simulink model "upr_1_2"  (R2019a)
settings: Solver=FixedStepAuto  StartTime=0.0  StopTime=100  FixedStep=0.1  RelTol=1e-3
settings Model: Creator=user1  LastModifiedBy=user1

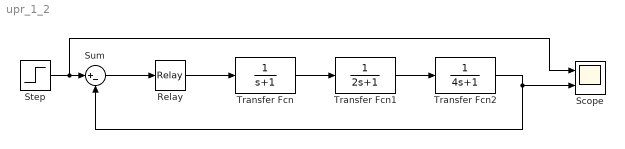
== system upr_1_2 ==
  Relay : Relay  OnOutputValue=2  OffOutputValue=-2
  Scope : Scope  NumInputPorts=2
  Step : Step  SampleTime=0
  Sum : Sum  Inputs=|+-
  Transfer Fcn : TransferFcn  Denominator=[1 1]
  Transfer Fcn1 : TransferFcn  Denominator=[2 1]
  Transfer Fcn2 : TransferFcn  Denominator=[4 1]
  wires:
  Sum/1 -> Relay/1
  Step/1 -> Scope/1, Sum/1
  Transfer Fcn/1 -> Transfer Fcn1/1
  Relay/1 -> Transfer Fcn/1
  Transfer Fcn2/1 -> Scope/2, Sum/2
  Transfer Fcn1/1 -> Transfer Fcn2/1
